simulink model "drone_v3"  (R2021a)
settings: configuration reference "ctrlConfigSet" (kept outside this file)
undefined symbols (not defined in the file or in its folder): uavParam
libraries: aerolibnav x2, simulink x2, shared6dof x1
settings Model: DataDictionary=pathFollowingData.sldd  Creator=The MathWorks, Inc.  LastModifiedBy=FusionLab
settings ConfigSetRef: SourceName=ctrlConfigSet

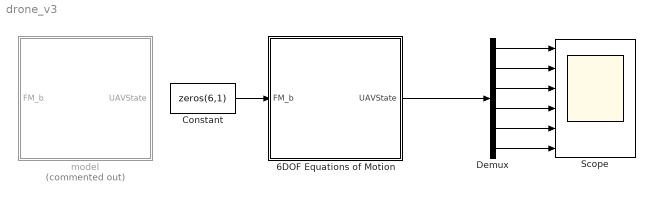
== system drone_v3 ==
  6DOF Equations of Motion : Subsystem  VariantControl=use_aerospace_blocks == 1
  Constant : Constant  Value=zeros(6,1)
  Demux : Demux  Outputs=6
  Scope : Scope  NumInputPorts=6
  model : Subsystem  Commented=on  VariantControl=use_aerospace_blocks == 1
  wires:
  Constant/1 -> 6DOF Equations of Motion/1(FM_b)
  6DOF Equations of Motion/1(UAVState) -> Demux/1
  Demux/1 -> Scope/1
  Demux/2 -> Scope/2
  Demux/3 -> Scope/3
  Demux/4 -> Scope/4
  Demux/5 -> Scope/5
  Demux/6 -> Scope/6

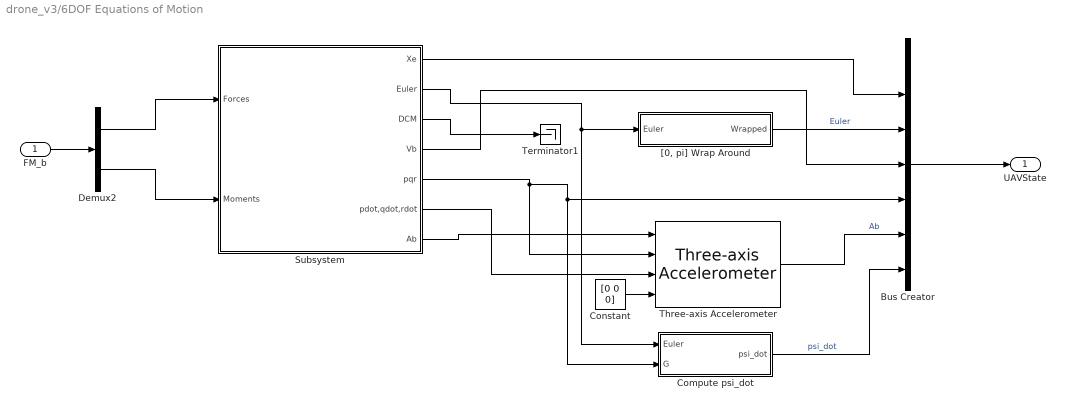
== system drone_v3/6DOF Equations of Motion ==
  FM_b : Inport
  Bus Creator : BusCreator  Inputs=7
  Compute psi_dot : Subsystem
  Constant : Constant  Value=[0 0 0]
      settings: AttributesFormatString=%<Value>
  Demux2 : Demux  Outputs=2
  Subsystem : Subsystem
  Terminator1 : Terminator
  Three-axis Accelerometer : aerolibnav/Three-axis Accelerometer  units=Metric (MKS)  acc=[0 0 0]  gtype=off  dtype_a=off  w_a=190  z_a=0.707  a_sf_cc=[1 0 0; 0 1 0; 0 0 1]  a_bias=[0 0 0]  a_Ts=0  a_rand=off  a_seeds=[23093 23094 23095]  a_pow=[0.001 0.001 0.001]  a_sat="[-inf  -inf  -inf  inf inf inf]"
      settings: SourceProductName=Aerospace Blockset
  "[0, pi] Wrap Around" : Subsystem
  UAVState : Outport  VectorParamsAs1DForOutWhenUnconnected=off
  wires:
  Three-axis Accelerometer/1 -> Bus Creator/6  "Ab"
  Constant/1 -> Three-axis Accelerometer/4
  "[0, pi] Wrap Around"/1(Wrapped) -> Bus Creator/3  "Euler"
  Bus Creator/1 -> UAVState/1
  FM_b/1 -> Demux2/1
  Compute psi_dot/1(psi_dot) -> Bus Creator/7  "psi_dot"
  Subsystem/5(pqr) -> Compute psi_dot/2(G), Bus Creator/5, Three-axis Accelerometer/2
  Subsystem/2(Euler) -> Compute psi_dot/1(Euler), "[0, pi] Wrap Around"/1(Euler)
  Demux2/1 -> Subsystem/1(Forces)
  Demux2/2 -> Subsystem/2(Moments)
  ? -> Bus Creator/1
  Subsystem/1(Xe) -> Bus Creator/2
  Subsystem/3(DCM) -> Terminator1/1
  Subsystem/4(Vb) -> Bus Creator/4
  Subsystem/6(pdot,qdot,rdot) -> Three-axis Accelerometer/3
  Subsystem/7(Ab) -> Three-axis Accelerometer/1

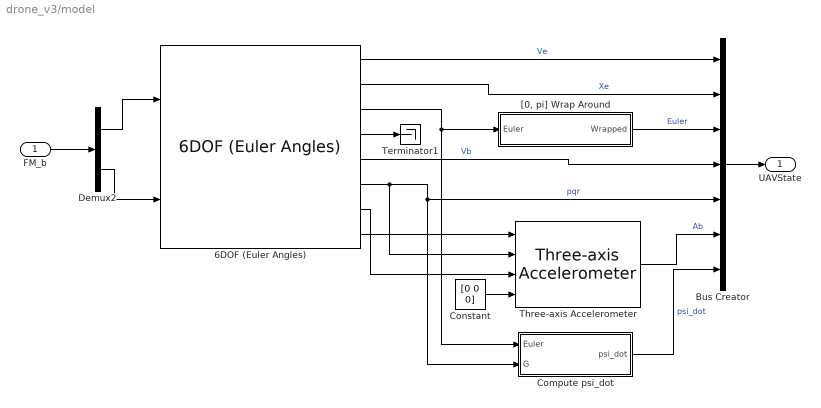
== system drone_v3/model ==
  FM_b : Inport
  6DOF (Euler Angles) : shared6dof/6DOF (Euler Angles)  units=Metric (MKS)  mtype=Fixed  rep=Euler Angles  xme_0=uavParam.ic.Pos_0.*[1; 1; -1]  Vm_0=uavParam.ic.Vb_0  eul_0=uavParam.ic.Euler_0  pm_0=uavParam.ic.PQR_0  mass_0=uavParam.geometry.mass  mass_e=0.5  mass_f=2.0  inertia=eye(3).*[uavParam.inertia.Ixx;uavParam.inertia.Iyy; uavParam.inertia.Izz]  inertia_e=eye(3)  inertia_f=2*eye(3)  k_quat=1.0  vre_flag=on  abi_flag=off  aMode=0  xme_statename=''  Vm_statename=''  eul_statename=''  quat_statename=''  pm_statename=''  mass_statename=''
      settings: SourceProductBaseCode=AE,PW,DR,MT,UV,VE
  Bus Creator : BusCreator  Inputs=7
  Compute psi_dot : Subsystem
  Constant : Constant  Value=[0 0 0]
      settings: AttributesFormatString=%<Value>
  Demux2 : Demux  Outputs=2
  Terminator1 : Terminator
  Three-axis Accelerometer : aerolibnav/Three-axis Accelerometer  units=Metric (MKS)  acc=[0 0 0]  gtype=off  dtype_a=off  w_a=190  z_a=0.707  a_sf_cc=[1 0 0; 0 1 0; 0 0 1]  a_bias=[0 0 0]  a_Ts=0  a_rand=off  a_seeds=[23093 23094 23095]  a_pow=[0.001 0.001 0.001]  a_sat="[-inf  -inf  -inf  inf inf inf]"
      settings: SourceProductName=Aerospace Blockset
  "[0, pi] Wrap Around" : Subsystem
  UAVState : Outport  VectorParamsAs1DForOutWhenUnconnected=off
  wires:
  Three-axis Accelerometer/1 -> Bus Creator/6  "Ab"
  Constant/1 -> Three-axis Accelerometer/4
  "[0, pi] Wrap Around"/1(Wrapped) -> Bus Creator/3  "Euler"
  6DOF (Euler Angles)/8 -> Three-axis Accelerometer/1
  6DOF (Euler Angles)/5 -> Bus Creator/4  "Vb"
  6DOF (Euler Angles)/2 -> Bus Creator/2  "Xe"
  6DOF (Euler Angles)/1 -> Bus Creator/1  "Ve"
  Bus Creator/1 -> UAVState/1
  6DOF (Euler Angles)/7 -> Three-axis Accelerometer/3
  6DOF (Euler Angles)/4 -> Terminator1/1
  6DOF (Euler Angles)/3 -> Compute psi_dot/1(Euler), "[0, pi] Wrap Around"/1(Euler)
  6DOF (Euler Angles)/6 -> Compute psi_dot/2(G), Bus Creator/5, Three-axis Accelerometer/2  "pqr"
  FM_b/1 -> Demux2/1
  Demux2/2 -> 6DOF (Euler Angles)/2
  Demux2/1 -> 6DOF (Euler Angles)/1
  Compute psi_dot/1(psi_dot) -> Bus Creator/7  "psi_dot"

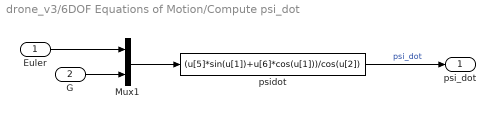
== system drone_v3/6DOF Equations of Motion/Compute psi_dot ==
  Euler : Inport
  G : Inport  Port=2
  Mux1 : Mux  Inputs=2
  psidot : Fcn  Expr=(u[5]*sin(u[1])+u[6]*cos(u[1]))/cos(u[2])
  psi_dot : Outport  Unit=rad/S  VectorParamsAs1DForOutWhenUnconnected=off
  wires:
  G/1 -> Mux1/2
  psidot/1 -> psi_dot/1  "psi_dot"
  Mux1/1 -> psidot/1
  Euler/1 -> Mux1/1

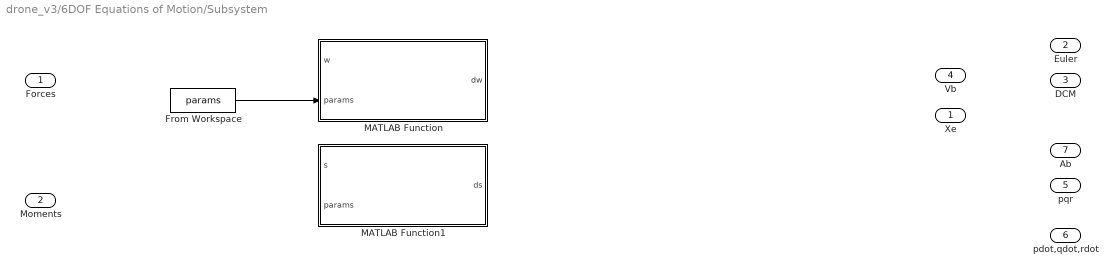
== system drone_v3/6DOF Equations of Motion/Subsystem ==
  Forces : Inport
  Moments : Inport  Port=2
  From Workspace : FromWorkspace  VariableName=params
  MATLAB Function : MATLAB Function  TreatAsAtomicUnit=on
  MATLAB Function1 : MATLAB Function  TreatAsAtomicUnit=on
  Xe : Outport
  Euler : Outport  Port=2
  DCM : Outport  Port=3
  Vb : Outport  Port=4
  pqr : Outport  Port=5
  pdot,qdot,rdot : Outport  Port=6
  Ab : Outport  Port=7
  wires:
  From Workspace/1 -> MATLAB Function/2(params)

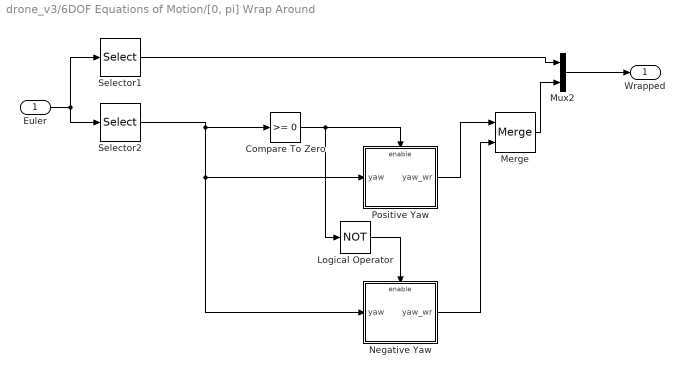
== system drone_v3/6DOF Equations of Motion/[0, pi] Wrap Around ==
  Euler : Inport
  Compare To Zero : simulink/Logic and Bit Operations/Compare To Zero  relop=>=  OutDataTypeStr=uint8  ZeroCross=off
  Logical Operator : Logic  Operator=NOT  AllPortsSameDT=off  OutDataTypeStr=boolean
  Merge : Merge  InitialOutput=0
  Mux2 : Mux  Inputs=2
  Negative Yaw : Subsystem
  Positive Yaw : Subsystem
  Selector1 : Selector  InputPortWidth=3  IndexOptions=Index vector (dialog)  Indices=[1 2]  OutputSizes=1
  Selector2 : Selector  InputPortWidth=3  IndexOptions=Index vector (dialog)  Indices=[3]  OutputSizes=1
  Wrapped : Outport  VectorParamsAs1DForOutWhenUnconnected=off
  wires:
  Negative Yaw/1(yaw_wr) -> Merge/2
  Positive Yaw/1(yaw_wr) -> Merge/1
  Merge/1 -> Mux2/2
  Logical Operator/1 -> Negative Yaw/Enable
  Compare To Zero/1 -> Logical Operator/1, Positive Yaw/Enable
  Selector2/1 -> Negative Yaw/1(yaw), Positive Yaw/1(yaw), Compare To Zero/1
  Mux2/1 -> Wrapped/1
  Selector1/1 -> Mux2/1
  Euler/1 -> Selector1/1, Selector2/1

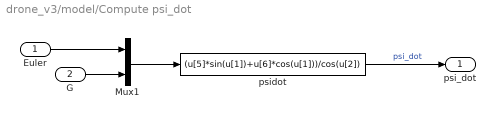
== system drone_v3/model/Compute psi_dot ==
  Euler : Inport
  G : Inport  Port=2
  Mux1 : Mux  Inputs=2
  psidot : Fcn  Expr=(u[5]*sin(u[1])+u[6]*cos(u[1]))/cos(u[2])
  psi_dot : Outport  Unit=rad/S  VectorParamsAs1DForOutWhenUnconnected=off
  wires:
  G/1 -> Mux1/2
  psidot/1 -> psi_dot/1  "psi_dot"
  Mux1/1 -> psidot/1
  Euler/1 -> Mux1/1

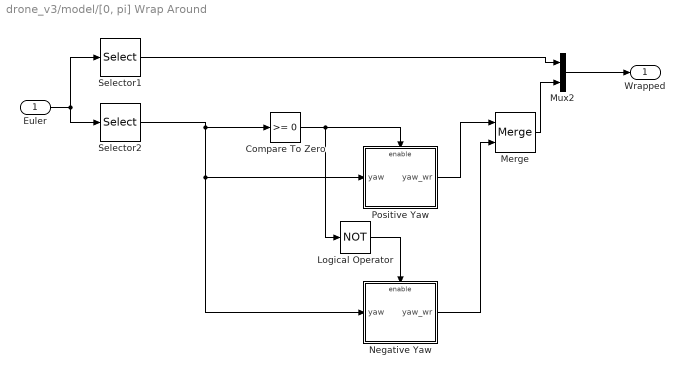
== system drone_v3/model/[0, pi] Wrap Around ==
  Euler : Inport
  Compare To Zero : simulink/Logic and Bit Operations/Compare To Zero  relop=>=  OutDataTypeStr=uint8  ZeroCross=off
  Logical Operator : Logic  Operator=NOT  AllPortsSameDT=off  OutDataTypeStr=boolean
  Merge : Merge  InitialOutput=0
  Mux2 : Mux  Inputs=2
  Negative Yaw : Subsystem
  Positive Yaw : Subsystem
  Selector1 : Selector  InputPortWidth=3  IndexOptions=Index vector (dialog)  Indices=[1 2]  OutputSizes=1
  Selector2 : Selector  InputPortWidth=3  IndexOptions=Index vector (dialog)  Indices=[3]  OutputSizes=1
  Wrapped : Outport  VectorParamsAs1DForOutWhenUnconnected=off
  wires:
  Negative Yaw/1(yaw_wr) -> Merge/2
  Positive Yaw/1(yaw_wr) -> Merge/1
  Merge/1 -> Mux2/2
  Logical Operator/1 -> Negative Yaw/Enable
  Compare To Zero/1 -> Logical Operator/1, Positive Yaw/Enable
  Selector2/1 -> Negative Yaw/1(yaw), Positive Yaw/1(yaw), Compare To Zero/1
  Mux2/1 -> Wrapped/1
  Selector1/1 -> Mux2/1
  Euler/1 -> Selector1/1, Selector2/1

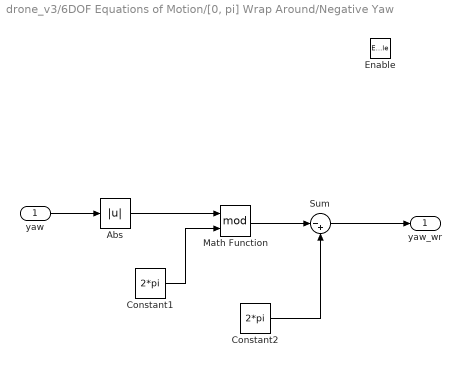
== system drone_v3/6DOF Equations of Motion/[0, pi] Wrap Around/Negative Yaw ==
  yaw : Inport
  Enable : EnablePort
  Abs : Abs
  Constant1 : Constant  Value=2*pi
      settings: AttributesFormatString=%<Value>
  Constant2 : Constant  Value=2*pi
      settings: AttributesFormatString=%<Value>
  Math Function : Math  Operator=mod  SignedPower=on  SaturateOnIntegerOverflow=on
  Sum : Sum  Inputs=|-+
  yaw_wr : Outport  VectorParamsAs1DForOutWhenUnconnected=off
  wires:
  Sum/1 -> yaw_wr/1
  Constant2/1 -> Sum/2
  Abs/1 -> Math Function/1
  Math Function/1 -> Sum/1
  Constant1/1 -> Math Function/2
  yaw/1 -> Abs/1

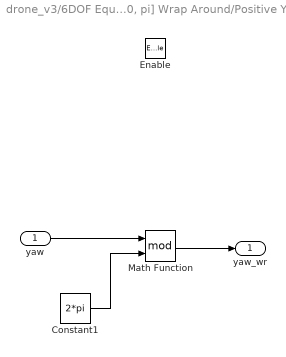
== system drone_v3/6DOF Equations of Motion/[0, pi] Wrap Around/Positive Yaw ==
  yaw : Inport
  Enable : EnablePort
  Constant1 : Constant  Value=2*pi
      settings: AttributesFormatString=%<Value>
  Math Function : Math  Operator=mod  SignedPower=on  SaturateOnIntegerOverflow=on
  yaw_wr : Outport  VectorParamsAs1DForOutWhenUnconnected=off
  wires:
  Math Function/1 -> yaw_wr/1
  Constant1/1 -> Math Function/2
  yaw/1 -> Math Function/1

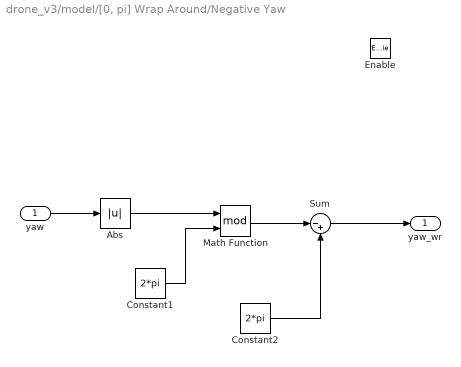
== system drone_v3/model/[0, pi] Wrap Around/Negative Yaw ==
  yaw : Inport
  Enable : EnablePort
  Abs : Abs
  Constant1 : Constant  Value=2*pi
      settings: AttributesFormatString=%<Value>
  Constant2 : Constant  Value=2*pi
      settings: AttributesFormatString=%<Value>
  Math Function : Math  Operator=mod  SignedPower=on  SaturateOnIntegerOverflow=on
  Sum : Sum  Inputs=|-+
  yaw_wr : Outport  VectorParamsAs1DForOutWhenUnconnected=off
  wires:
  Sum/1 -> yaw_wr/1
  Constant2/1 -> Sum/2
  Abs/1 -> Math Function/1
  Math Function/1 -> Sum/1
  Constant1/1 -> Math Function/2
  yaw/1 -> Abs/1

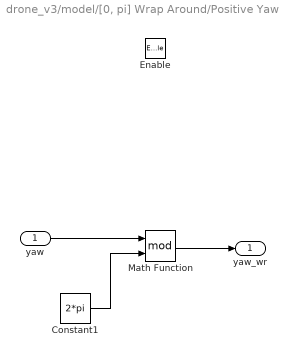
== system drone_v3/model/[0, pi] Wrap Around/Positive Yaw ==
  yaw : Inport
  Enable : EnablePort
  Constant1 : Constant  Value=2*pi
      settings: AttributesFormatString=%<Value>
  Math Function : Math  Operator=mod  SignedPower=on  SaturateOnIntegerOverflow=on
  yaw_wr : Outport  VectorParamsAs1DForOutWhenUnconnected=off
  wires:
  Math Function/1 -> yaw_wr/1
  Constant1/1 -> Math Function/2
  yaw/1 -> Math Function/1

== matlab function drone_v3/6DOF Equations of Motion/Subsystem/MATLAB Function1 ==
  data: ds output; s input; params input
function ds = PositionDynamics_v1(s,params)

    %inizializzazione
    ds=zeros(size(s));
    %position, linear velocity
    ned=s(1:3);
    velocity=s(4:6);

    xdot=velocity(3)*(sin(params.eul(1))*sin(params.eul(3))+cos(params.eul(1))*cos(params.eul(3))*sin(params.eul(2)))-velocity(2)*(cos(params.eul(1))*sin(params.eul(3))-cos(params.eul(3))*sin(params.eul(1))*sin(params.eul(2)))+velocity(1)*(cos(params.eul(3))*cos(params.eul(2)));
    ydot=velocity(2)*(cos(params.eul(1))*cos(params.eul(3))+sin(params.eul(1))*sin(params.eul(3))*sin(params.eul(2)))-velocity(3)*(cos(params.eul(3))*sin(params.eul(1))-cos(params.eul(1))*sin(params.eul(3))*sin(params.eul(2)))+velocity(1)*(cos(params.eul(2))*sin(params.eul(3)));
    zdot=velocity(3)*(cos(params.eul(1))*cos(params.eul(2)))-velocity(1)*sin(params.eul(2))+velocity(2)*(cos(params.eul(2))*sin(params.eul(1)));

    udot=params.omega(3)*velocity(2)-params.omega(2)*velocity(3)-params.g*sin(params.eul(2));
    vdot=params.omega(1)*velocity(3)-params.omega(3)*velocity(1)+params.g*sin(params.eul(1))*cos(params.eul(2));
    wdot=params.omega(2)*velocity(1)-params.omega(1)*velocity(2)+params.g*cos(params.eul(2))*cos(params.eul(1));
    ds=[xdot;ydot;zdot;udot;vdot;wdot];
end

== matlab function drone_v3/6DOF Equations of Motion/Subsystem/MATLAB Function ==
  data: dw output; w input; params input
function dw = AttitudeDynamics_v1(w,params)



% Initialize integration vectors and parameters

dw = zeros(size(w));


% Extract attitude, angular velocity 
q =  w(1:4);
omega= w(5:7);


%%%%%%%%%%%%%%%%%% Attitude Kinematics Equations (Quaternions) %%%%%%%%%%%%%%%%%%
Om = [0, -omega(1), -omega(2), -omega(3);
    omega(1), 0, omega(3), -omega(2);
    omega(2), -omega(3), 0, omega(1);
    omega(3), omega(2), -omega(1), 0];
dw(1:4,1) = 0.5*Om*q;

omega_thrust = 0.159155*params.omegaThrust;
Mx=params.l*params.b*(omega_thrust(2)^2-omega_thrust(4)^2);
My=params.l*params.b*(omega_thrust(1)^2-omega_thrust(3)^2);
Mz=params.d*(omega_thrust(1)^2-omega_thrust(2)^2+omega_thrust(3)^2-omega_thrust(4)^2);



pdot=(Mx/params.I(1,1))-omega(2)*omega(3)*(params.I(3,3)-params.I(2,2))/params.I(1,1);
qdot=(My/params.I(1,1))-omega(1)*omega(3)*(params.I(1,1)-params.I(3,3))/params.I(2,2);
rdot=(Mz/params.I(3,3));
dw(5:7)=[pdot; qdot; rdot];

end
